simulink model "Real_World_1m"  (R2021a)
settings: Solver=FixedStepDiscrete  StartTime=0.0  StopTime=10.0  FixedStep=0.01  RelTol=1e-3
values from neighbouring files (symbols this model uses):
  ticksPerRot = 20    [robotParameters.m]
  wheelR = 0.031    [robotParameters.m]
undefined symbols (not defined in the file or in its folder): InputPWM, WheelSpeed
libraries: arduinolib x6, spsEdgeDetectorLib x2, mobileRoboticsTrainingLib x1
settings Model: SILPILModeSetting=veronly  EnablePacing=on  ExtModeTrigDuration=2  Creator=Boitumelo  LastModifiedBy=akhil
settings SolverCC: AlgebraicLoopSolver=TrustRegion
settings OptimizationCC: EnhancedBackFolding=on  PassReuseOutputArgsAs=Individual arguments  ZeroExternalMemoryAtStartup=off  ZeroInternalMemoryAtStartup=off  MaxStackSize=64  OptimizeBlockOrder=speed  DifferentSizesBufferReuse=on  OptimizationCustomize=off  EfficientTunableParamExpr=on
settings DebuggingCC: ParameterTunabilityLossMsg=error
settings HardwareCC: ProdBitPerInt=16  ProdBitPerPointer=16  ProdBitPerSizeT=16  ProdBitPerPtrDiffT=16  ProdLargestAtomicFloat=None  ProdWordSize=8  ProdHWDeviceType=Atmel->AVR
settings SFSimCC: MATLABDynamicMemAlloc=off
settings RTWCC: SystemTargetFile=ert.tlc  HardwareBoard=Arduino Leonardo  TemplateMakefile=ert_default_tmf  Toolchain=Arduino AVR
settings CodeAppCC: ForceParamTrailComments=on  IgnoreCustomStorageClasses=off  OperatorAnnotations=on  SimulinkDataObjDesc=on  SFDataObjDesc=on  InsertBlockDesc=on
settings ERTTargetCC: SupportContinuousTime=on  SupportVariableSizeSignals=on  ExtModeTransport=6  ExtModeStaticAllocSize=250  ExtModeMexFile=ext_serial_win32_comm_leonardo

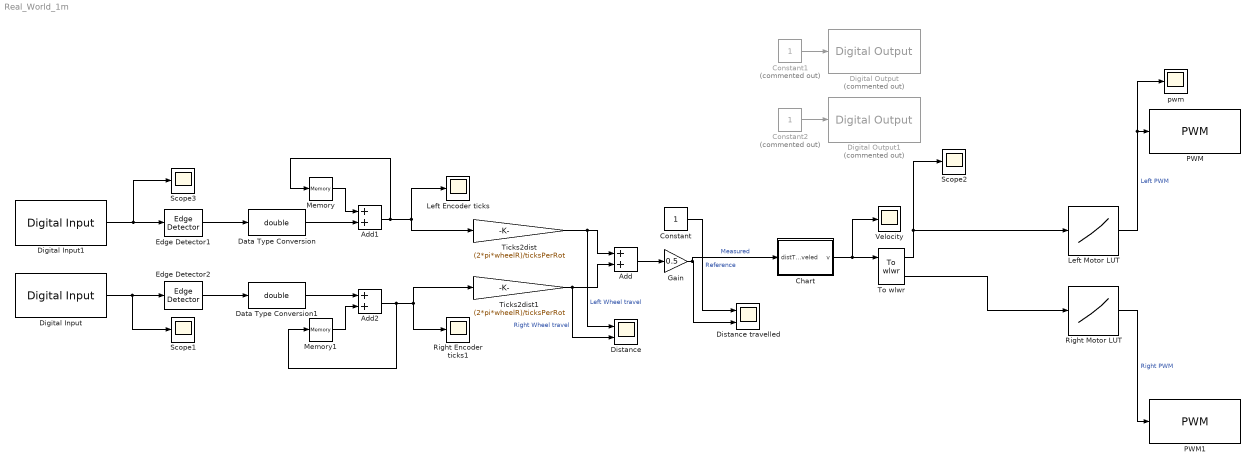
== system Real_World_1m ==
  Add : Sum
  Add1 : Sum
  Add2 : Sum
  Chart : Stateflow chart  TreatAsAtomicUnit=on
  Constant : Constant
  Constant1 : Constant  Commented=on
  Constant2 : Constant  Commented=on
  Data Type Conversion : DataTypeConversion  OutDataTypeStr=double
  Data Type Conversion1 : DataTypeConversion  OutDataTypeStr=double
  Digital Input : arduinolib/Digital Input  pinNumber=3  mode=Default  Direction=input  SampleTime=0.01  blockPlatform=arduino
  Digital Input1 : arduinolib/Digital Input  pinNumber=2  mode=Default  Direction=input  SampleTime=0.01  blockPlatform=arduino
  Digital Output : arduinolib/Digital Output  Commented=on  pinNumber=4  Direction=output  blockPlatform=arduino
  Digital Output1 : arduinolib/Digital Output  Commented=on  pinNumber=7  Direction=output  blockPlatform=arduino
  Distance : Scope  NumInputPorts=2
  Distance travelled : Scope  NumInputPorts=2
  Edge Detector1 : spsEdgeDetectorLib/Edge Detector  model=Either  ic=0  Ts=0
      settings: SourceProductBaseCode=PS
  Edge Detector2 : spsEdgeDetectorLib/Edge Detector  model=Either  ic=0  Ts=0
      settings: SourceProductBaseCode=PS
  Gain : Gain  Gain=0.5
  Left Encoder ticks : Scope
  Left Motor LUT : Lookup_n-D  NumberOfTableDimensions=1  BreakpointsForDimension1=WheelSpeed  Table=InputPWM  InterpMethod=Nearest  ExtrapMethod=Clip  InternalRulePriority=Speed  RndMeth=Simplest  InputSameDT=on
  Memory : Memory
  Memory1 : Memory
  PWM : arduinolib/PWM  pinNumber=5  frequencyType=Default  desiredFrequency=490.2  achievableFrequency=490.2
  PWM1 : arduinolib/PWM  pinNumber=6  frequencyType=Default  desiredFrequency=490.2  achievableFrequency=490.2
  Right Encoder ticks1 : Scope
  Right Motor LUT : Lookup_n-D  NumberOfTableDimensions=1  BreakpointsForDimension1=WheelSpeed  Table=InputPWM  InterpMethod=Nearest  ExtrapMethod=Clip  InternalRulePriority=Speed  RndMeth=Simplest  InputSameDT=on
  Scope1 : Scope
  Scope2 : Scope
  Scope3 : Scope
  Ticks2dist : Gain  Gain=(2*pi*wheelR)/ticksPerRot
  Ticks2dist1 : Gain  Gain=(2*pi*wheelR)/ticksPerRot
  To wlwr : mobileRoboticsTrainingLib/To wlwr  axleLength=0.1  wheelR=0.05
  Velocity : Scope
  pwm : Scope
  wires:
  Right Motor LUT/1 -> PWM1/1  "Right PWM"
  Left Motor LUT/1 -> pwm/1, PWM/1  "Left PWM"
  To wlwr/1 -> Left Motor LUT/1, Scope2/1
  Add/1 -> Gain/1
  Gain/1 -> Chart/1(distTraveled), Distance travelled/2  "Measured"
  Ticks2dist/1 -> Distance/1, Add/1  "Left Wheel travel"
  Constant/1 -> Distance travelled/1  "Reference"
  Ticks2dist1/1 -> Distance/2, Add/2  "Right Wheel travel"
  Constant1/1 -> Digital Output/1
  Constant2/1 -> Digital Output1/1
  Digital Input1/1 -> Scope3/1, Edge Detector1/1
  Digital Input/1 -> Scope1/1, Edge Detector2/1
  Edge Detector1/1 -> Data Type Conversion/1
  Edge Detector2/1 -> Data Type Conversion1/1
  Data Type Conversion/1 -> Add1/2
  Data Type Conversion1/1 -> Add2/1
  Memory/1 -> Add1/1
  Memory1/1 -> Add2/2
  Add1/1 -> Memory/1, Ticks2dist/1, Left Encoder ticks/1
  Add2/1 -> Memory1/1, Ticks2dist1/1, Right Encoder ticks1/1
  Chart/1(v) -> Velocity/1, To wlwr/1
  To wlwr/2 -> Right Motor LUT/1

== stateflow chart Real_World_1m/Chart ==
  state MoveForward
    entry:
    v = 0.1
  state Stop
    entry:
    v = 0
  (default) -> MoveForward : % Start
  MoveForward -> Stop : [distTraveled >= 1]
  data: distTraveled input; v output
